simulink model "gravity"  (R2024a)
settings: configuration reference "autoCodeSILConfigurationParams" (kept outside this file)
undefined symbols (not defined in the file): stepSize_s
settings Model: Creator=GTAR  LastModifiedBy=jerem
settings ConfigSetRef: SourceName=autoCodeSILConfigurationParams  SourceLocation=Base Workspace

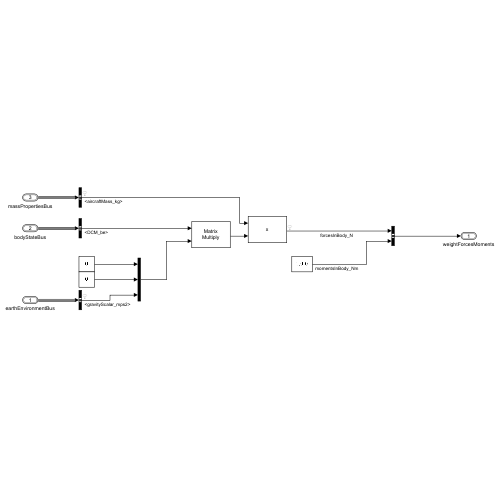
[thumbnail: Simulink's stored preview of the top-level diagram]
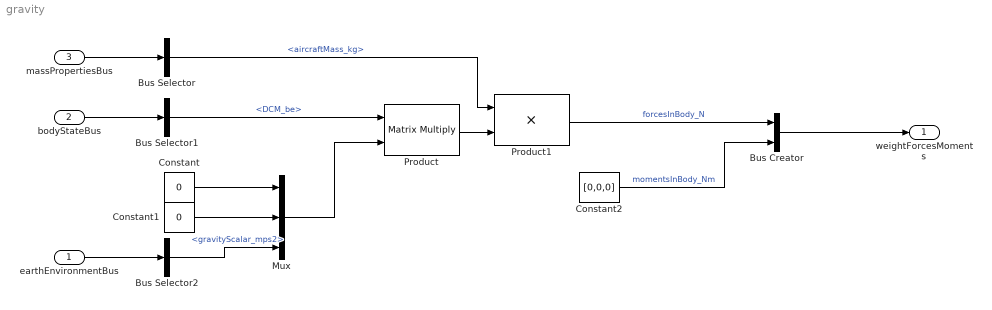
== system gravity ==
  earthEnvironmentBus : Inport  OutDataTypeStr=Bus: EarthEnvironmentBus
  bodyStateBus : Inport  Port=2  OutDataTypeStr=Bus: BodyStateBus
  massPropertiesBus : Inport  Port=3  OutDataTypeStr=Bus: MassPropertiesBus
  Bus Creator : BusCreator  Inputs=2  OutDataTypeStr=Bus: ComponentForcesMomentsBus  NonVirtualBus=on
  Bus Selector : BusSelector  OutputSignals=aircraftMass_kg
  Bus Selector1 : BusSelector  OutputSignals=DCM_be
  Bus Selector2 : BusSelector  OutputSignals=gravityScalar_mps2
  Constant : Constant  Value=0  SampleTime=stepSize_s
  Constant1 : Constant  Value=0  SampleTime=stepSize_s
  Constant2 : Constant  Value=[0,0,0]  SampleTime=stepSize_s
  Mux : Mux  Inputs=3
  Product : Product  Multiplication=Matrix(*)
  Product1 : Product
  weightForcesMoments : Outport  OutDataTypeStr=Bus: ComponentForcesMomentsBus
  wires:
  Constant/1 -> Mux/1
  bodyStateBus/1 -> Bus Selector1/1
  Product/1 -> Product1/2
  Mux/1 -> Product/2
  Constant1/1 -> Mux/2
  massPropertiesBus/1 -> Bus Selector/1
  Bus Selector/1 -> Product1/1  "<aircraftMass_kg>"
  Bus Selector1/1 -> Product/1  "<DCM_be>"
  earthEnvironmentBus/1 -> Bus Selector2/1
  Bus Selector2/1 -> Mux/3  "<gravityScalar_mps2>"
  Product1/1 -> Bus Creator/1  "forcesInBody_N"
  Constant2/1 -> Bus Creator/2  "momentsInBody_Nm"
  Bus Creator/1 -> weightForcesMoments/1
